simulink model "motor_position_ctrl"  (R2020b)
settings: Solver=VariableStepAuto  StartTime=0.0  StopTime=10.0  RelTol=1e-3
settings Model: Creator=ADMIN  LastModifiedBy=ADMIN

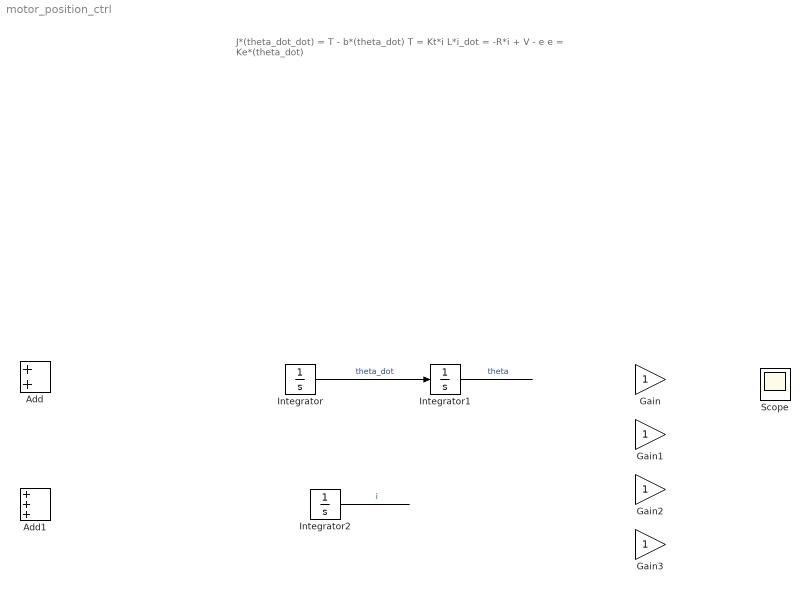
== system motor_position_ctrl ==
  note: J*(theta_dot_dot) = T - b*(theta_dot)
      |
      | T = Kt*i
      |
      | L*i_dot = -R*i + V - e
      |
      | e = Ke*(theta_dot)
  Add : Sum
  Add1 : Sum  Inputs=+++
  Gain{,1..3} (4 alike) : Gain
  Integrator : Integrator
  Integrator1 : Integrator
  Integrator2 : Integrator
  Scope : Scope
  wires:
  Integrator/1 -> Integrator1/1  "theta_dot"
  ? -> Integrator/1  "theta_dot_dot"
  Integrator1/1 -> ?  "theta"
  Integrator2/1 -> ?  "i"
  ? -> Integrator2/1  "i_dot"
